simulink model "ParameterEstimationSimpleDCmotor"  (R2018b)
settings: Solver=ode15s  StartTime=0.0  StopTime=8  RelTol=1e-3
model workspace (MAT data in the model file):
  ParameterEstimationSimpleDCmotor_spesession : sldodialogs.data.SessionData (value not decoded)
values from neighbouring files (symbols this model uses):
  B = 0.01    [dc_motor_script.m]    (also in values_03.mat = 0.0197154970974)
  K = 1    [dc_motor_script.m]    (also in values_03.mat = 0.824871094407)
  R = 10    [dc_motor_script.m]    (also in values_03.mat = 7.97590597357)
  rpm_to_rads = 0.104719755    [dc_motor_script.m]
libraries: fl_lib x12, nesl_utility x6, elec_lib x2
settings Model: Creator=EDU_UGEX_7219  LastModifiedBy=EDU_UGEX_7219
settings DataIOCC: ExternalInput=[ReversePortTime, ReversePortVoltage]  LoadExternalInput=on  SaveFormat=Array

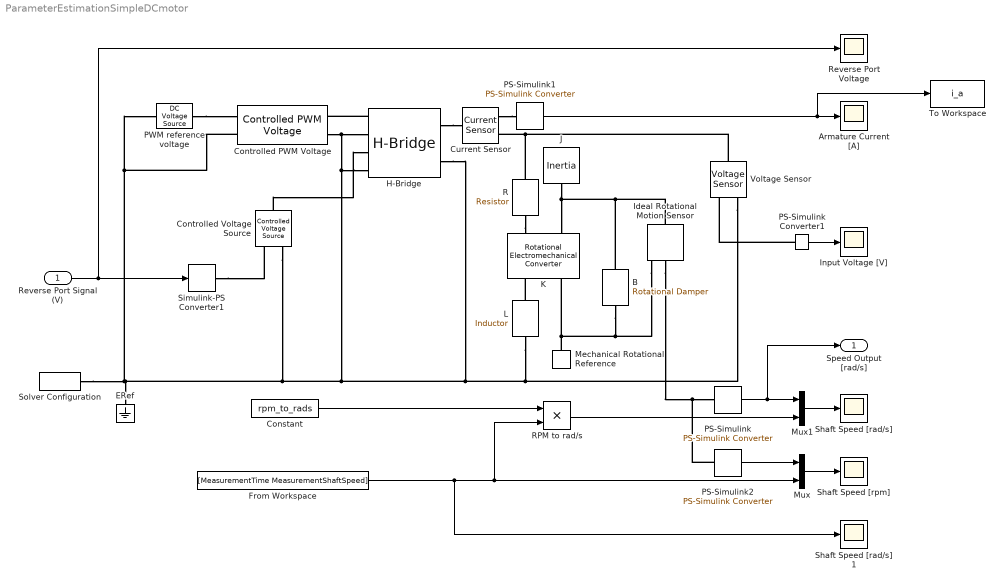
== system ParameterEstimationSimpleDCmotor ==
  Reverse Port Signal (V) : Inport
  "Armature Current [A] " : Scope
  B : fl_lib/Mechanical/Rotational Elements/Rotational Damper  D=B N*m/(rad/s)  w_specify=off  w_priority=None  w=0 rad/s  w_nominal_specify=off  w_nominal_unit=rad/s  w_nominal_value=1  t_specify=off  t_priority=None  t=0 N*m  t_nominal_specify=off  t_nominal_unit=N*m  t_nominal_value=1
  Constant : Constant  Value=rpm_to_rads
  Controlled Voltage Source : fl_lib/Electrical/Electrical Sources/Controlled Voltage Source
  Controlled PWM Voltage : elec_lib/Actuators & Drivers/Drivers/Controlled PWM Voltage  F=4000 Hz  TD=0 s  pulse_width_offset=0 s  pulse_min=0 s  Vmin=0 V  Vmax=5 V  Vm=5 V  pwm_or_av=2  event_type=1  sample_time=1e-6 s  u_min=0  u_max=1
      settings: SourceProductName=Simscape Electronics  SourceProductBaseCode=SN
  "Current Sensor " : fl_lib/Electrical/Electrical Sensors/Current Sensor
      settings: SourceProductName=Foundation Library
  ERef : fl_lib/Electrical/Electrical Elements/Electrical Reference
      settings: SourceProductName=Foundation Library
  From Workspace : FromWorkspace  VariableName=[MeasurementTime MeasurementShaftSpeed]  SampleTime=0
  H-Bridge : elec_lib/Actuators & Drivers/Drivers/H-Bridge  Venable=2.5 V  Vmax=5 V  Vreverse=2.5 V  Vbrake=2.5 V  Vm=12 V  pwm_or_av=2  discontinuous=0  freewheeling_mode=1  freewheeling_mode_disc=1  Ron=0.1 Ohm  Don=0.1 Ohm  Rload=3.38+0.1 Ohm  Lload=1e-5 H  F=4 kHz  thermal_mass=100 J/K  initial_temperature=298.15 K  Ron2=0.1 Ohm  Don2=0.05 Ohm  Tmeas=298.15 K  Tmeas2=398.15 K
      settings: SourceProductName=Simscape Electronics  SourceProductBaseCode=SN
  Ideal Rotational Motion Sensor : fl_lib/Mechanical/Mechanical Sensors/Ideal Rotational Motion Sensor  offset=0 deg
      settings: SourceProductName=Foundation Library
  "Input Voltage [V] " : Scope
  J : fl_lib/Mechanical/Rotational Elements/Inertia  inertia=J kg*m^2  w_specify=off  w_priority=High  w=0 rad/s  w_nominal_specify=off  w_nominal_unit=rad/s  w_nominal_value=1  t_specify=off  t_priority=None  t=0 N*m  t_nominal_specify=off  t_nominal_unit=N*m  t_nominal_value=1
  K : fl_lib/Electrical/Electrical Elements/Rotational Electromechanical Converter  K=K V/(rad/s)  i_specify=off  i_priority=None  i=0 A  i_nominal_specify=off  i_nominal_unit=A  i_nominal_value=1  v_specify=off  v_priority=None  v=0 V  v_nominal_specify=off  v_nominal_unit=V  v_nominal_value=1  t_specify=off  t_priority=None  t=0 N*m  t_nominal_specify=off  t_nominal_unit=N*m  t_nominal_value=1  w_specify=off  w_priority=None  w=0 rad/s  w_nominal_specify=off  w_nominal_unit=rad/s  w_nominal_value=1
      settings: SourceProductName=Simscape
  L : fl_lib/Electrical/Electrical Elements/Inductor  l=L H  r=0 Ohm  g=1e-9 1/Ohm  i_specify=off  i_priority=None  i=0 A  i_nominal_specify=off  i_nominal_unit=A  i_nominal_value=1  v_specify=off  v_priority=None  v=0 V  v_nominal_specify=off  v_nominal_unit=V  v_nominal_value=1  i_L_specify=off  i_L_priority=High  i_L=0 A  i_L_nominal_specify=off  i_L_nominal_unit=A  i_L_nominal_value=1
  Mechanical Rotational Reference : fl_lib/Mechanical/Rotational Elements/Mechanical Rotational Reference
  Mux : Mux  Inputs=2
  Mux1 : Mux  Inputs=2
  PS-Simulink : nesl_utility/PS-Simulink Converter  PhysicalDomain=network_engine_domain  SubClassName=ps_output  LeftPortType=input  RightPortType=output  PseudoPeriodic=off  Frequencies=[]  Unit=rad/s  AffineConversion=off
  PS-Simulink Converter1 : nesl_utility/PS-Simulink Converter  PhysicalDomain=network_engine_domain  SubClassName=ps_output  LeftPortType=input  RightPortType=output  PseudoPeriodic=off  Frequencies=[]  Unit=V  AffineConversion=off
  PS-Simulink1 : nesl_utility/PS-Simulink Converter  PhysicalDomain=network_engine_domain  SubClassName=ps_output  LeftPortType=input  RightPortType=output  PseudoPeriodic=off  Frequencies=[]  Unit=A  AffineConversion=off
  PS-Simulink2 : nesl_utility/PS-Simulink Converter  PhysicalDomain=network_engine_domain  SubClassName=ps_output  LeftPortType=input  RightPortType=output  PseudoPeriodic=off  Frequencies=[]  Unit=rpm  AffineConversion=off
  PWM reference voltage : fl_lib/Electrical/Electrical Sources/DC Voltage Source  v0=5 V
      settings: SourceProductName=Foundation Library
  R : fl_lib/Electrical/Electrical Elements/Resistor  R=R Ohm  i_specify=off  i_priority=None  i=0 A  i_nominal_specify=off  i_nominal_unit=A  i_nominal_value=1  v_specify=off  v_priority=None  v=0 V  v_nominal_specify=off  v_nominal_unit=V  v_nominal_value=1
  RPM to rad/s : Product  Inputs=**
  Reverse Port Voltage : Scope
  "Shaft Speed [rad/s] " : Scope
  Shaft Speed [rad/s] 1 : Scope
  Shaft Speed [rpm] : Scope
  Simulink-PS Converter1 : nesl_utility/Simulink-PS Converter  PhysicalDomain=network_engine_domain  SubClassName=ps_input  LeftPortType=input  RightPortType=output  PseudoPeriodic=off  Frequencies=[]  NoiseDistribution=none  NoiseParameters=[]  Unit=1  AffineConversion=off  FilteringAndDerivatives=zero  SimscapeFilterOrder=1  InputFilterTimeConstant=.001  UdotUserProvided=0
  Solver Configuration : nesl_utility/Solver Configuration  PhysicalDomain=network_engine_domain  SubClassName=solver  LeftPortType=input  RightPortType=generic  Tones=[]  Harmonics=[]  SimulateNoise=off  Profile=off  UseLocalSampling=off  EnableSwitchedLinearOptims=on  FrequencyDomain=off  UseCCode=off  RelTol=0.001  AbsTol=1e-06  MinStep=1e-09  ToWorkspace=off  RevertToSquareIcSolve=off  NumHomotopyIterations=100  PhasorMode=off  PhasorModeNumHarmonics=1  DoDC=off  ResidualTolerance=1e-9  UseLocalSolver=off  LocalSolverChoice=NE_BACKWARD_EULER_ADVANCER  LocalSolverSampleTime=.001  DoFixedCost=off  MaxNonlinIter=3  MaxModeIter=2  LinearAlgebra=auto  EquationFormulation=NE_TIME_EF  DelaysMemoryBudget=1024  AutomaticFiltering=on  FilteringTimeConstant=0.001  PartitionStorageMethod=AS_NEEDED  PartitionMemoryBudget=1024
  To Workspace : ToWorkspace  VariableName=i_a  SampleTime=-1
  "Voltage Sensor " : fl_lib/Electrical/Electrical Sensors/Voltage Sensor
  "Speed Output [rad/s] " : Outport
  wires:
  PS-Simulink Converter1/1 -> "Input Voltage [V] "/1
  PS-Simulink1/1 -> To Workspace/1, "Armature Current [A] "/1
  Reverse Port Signal (V)/1 -> Simulink-PS Converter1/1, Reverse Port Voltage/1
  Mux/1 -> Shaft Speed [rpm]/1
  PS-Simulink2/1 -> Mux/1
  From Workspace/1 -> Shaft Speed [rad/s] 1/1, RPM to rad/s/2, Mux/2
  Constant/1 -> RPM to rad/s/1
  RPM to rad/s/1 -> Mux1/2
  Mux1/1 -> "Shaft Speed [rad/s] "/1
  PS-Simulink/1 -> "Speed Output [rad/s] "/1, Mux1/1
  connections:
  H-Bridge/LConn4 -- H-Bridge/LConn2 -- Controlled PWM Voltage/RConn2 -- L/RConn1 -- "Voltage Sensor "/RConn2 -- H-Bridge/RConn2 -- Controlled Voltage Source/RConn2 -- Solver Configuration/RConn1 -- PWM reference voltage/RConn1 -- Controlled PWM Voltage/LConn2 -- ERef/LConn1
  "Voltage Sensor "/LConn1 -- R/LConn1 -- "Current Sensor "/RConn2
  PS-Simulink Converter1/LConn1 -- "Voltage Sensor "/RConn1
  PWM reference voltage/LConn1 -- Controlled PWM Voltage/LConn1
  H-Bridge/LConn1 -- Controlled PWM Voltage/RConn1
  "Current Sensor "/RConn1 -- PS-Simulink1/LConn1
  Ideal Rotational Motion Sensor/RConn2 -- PS-Simulink2/LConn1 -- PS-Simulink/LConn1
  H-Bridge/RConn1 -- "Current Sensor "/LConn1
  Controlled Voltage Source/LConn1 -- H-Bridge/LConn3
  Simulink-PS Converter1/RConn1 -- Controlled Voltage Source/RConn1
  B/RConn1 -- Ideal Rotational Motion Sensor/RConn1 -- Mechanical Rotational Reference/LConn1 -- K/RConn2
  R/RConn1 -- K/LConn1
  J/LConn1 -- Ideal Rotational Motion Sensor/LConn1 -- B/LConn1 -- K/LConn2
  L/LConn1 -- K/RConn1
